simulink model "Sim_Ideal"  (R2017b)
settings: Solver=FixedStepAuto  StartTime=0.0  StopTime=t_total  FixedStep=1e-6  MaxStep=1e-4  RelTol=1e-3
values from neighbouring files (symbols this model uses):
  C21 = 100e-6    (= 0.0001)    [main_simu.m]
  C22 = 100e-6    (= 0.0001)    [main_simu.m]
  C23 = 220e-6    (= 0.00022)    [main_simu.m]
  C24 = 330e-6    (= 0.00033)    [main_simu.m]
  L41 = 10e-3    (= 0.01)    [main_simu.m]
  L42 = 10e-3    (= 0.01)    [main_simu.m]
  L43 = 10e-3    (= 0.01)    [main_simu.m]
  L44 = 100e-3    (= 0.1)    [main_simu.m]
  L61 = 1e-3    (= 0.001)    [main_simu.m]
  L62 = 1e-3    (= 0.001)    [main_simu.m]
  L63 = 1e-3    (= 0.001)    [main_simu.m]
  L64 = 1e-3    (= 0.001)    [main_simu.m]
  R21 = 2e3    (= 2000)    [main_simu.m]
  R22 = 1e3    (= 1000)    [main_simu.m]
  R23 = 500    [main_simu.m]
  R24 = 300    [main_simu.m]
  R31 = 2.5    [main_simu.m]
  R32 = 5    [main_simu.m]
  R33 = 8    [main_simu.m]
  R34 = 10    [main_simu.m]
  R41 = 10    [main_simu.m]
  R42 = 20    [main_simu.m]
  R43 = 30    [main_simu.m]
  R44 = 30    [main_simu.m]
  R51 = 10    [main_simu.m]
  R52 = 12    [main_simu.m]
  R53 = 15    [main_simu.m]
  R54 = 20    [main_simu.m]
  R61 = 10    [main_simu.m]
  R62 = 5    [main_simu.m]
  R63 = 30    [main_simu.m]
  R64 = 105    [main_simu.m]
  R71 = 5    [main_simu.m]
  R72 = 10    [main_simu.m]
  R73 = 20    [main_simu.m]
  R74 = 50    [main_simu.m]
  sim_off = sim_on    [double.m]    (also in fourfold.m; individual.m; main_simu.m; quintuple.m)
  sim_on = 50*ones(1,28)    [double.m]    (also in fourfold.m; individual.m; main_simu.m = 50*ones(1,num_cargas); quintuple.m)
  Valpha5 = 60    [main_simu.m]
  Valpha6 = 60    [main_simu.m]
undefined symbols (not defined in the file or in its folder): J, Laq, Lse, R, Ra, Rse, SEIP4, SEVP4, wm0, wmo
libraries: powerlib x204, simulink x72
(part 1 of 2)
settings Model: Creator=USUARIO  LastModifiedBy=USUARIO
settings SolverCC: DecoupledContinuousIntegration=on

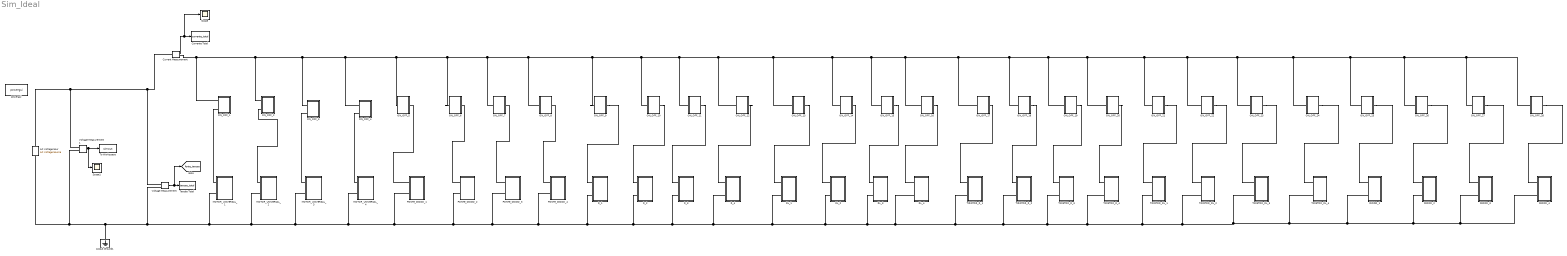
== system Sim_Ideal ==
  AC Voltage Sour : powerlib/Electrical Sources/AC Voltage Source  Amplitude=180  Phase=0  Frequency=60  SampleTime=0  Measurements=None  BusType=swing  Pref=10e3  Qref=0  Qmin=-inf  Qmax=+inf
  Corrente Total : ToWorkspace  VariableName=corrente_total  SampleTime=-1
  Current Measurement : powerlib/Measurements/Current Measurement  PhasorSimulation=off  OutputType=Complex  PSBequivalent=0
  DIODO_1 : Subsystem
  DIODO_2 : Subsystem
  DIODO_3 : Subsystem
  DIODO_4 : Subsystem
  MOTOR_UNIVERSAL_1 : Subsystem
  MOTOR_UNIVERSAL_2 : Subsystem
  MOTOR_UNIVERSAL_3 : Subsystem
  MOTOR_UNIVERSAL_4 : Subsystem
  ON_OFF_1 : Subsystem
  ON_OFF_10 : Subsystem
  ON_OFF_11 : Subsystem
  ON_OFF_12 : Subsystem
  ON_OFF_13 : Subsystem
  ON_OFF_14 : Subsystem
  ON_OFF_15 : Subsystem
  ON_OFF_16 : Subsystem
  ON_OFF_17 : Subsystem
  ON_OFF_18 : Subsystem
  ON_OFF_19 : Subsystem
  ON_OFF_2 : Subsystem
  ON_OFF_20 : Subsystem
  ON_OFF_21 : Subsystem
  ON_OFF_22 : Subsystem
  ON_OFF_23 : Subsystem
  ON_OFF_24 : Subsystem
  ON_OFF_25 : Subsystem
  ON_OFF_26 : Subsystem
  ON_OFF_27 : Subsystem
  ON_OFF_28 : Subsystem
  ON_OFF_3 : Subsystem
  ON_OFF_4 : Subsystem
  ON_OFF_5 : Subsystem
  ON_OFF_6 : Subsystem
  ON_OFF_7 : Subsystem
  ON_OFF_8 : Subsystem
  ON_OFF_9 : Subsystem
  PONTE_DIODO_1 : Subsystem
  PONTE_DIODO_2 : Subsystem
  PONTE_DIODO_3 : Subsystem
  PONTE_DIODO_4 : Subsystem
  RL_1 : Subsystem
  RL_2 : Subsystem
  RL_3 : Subsystem
  RL_4 : Subsystem
  R_1 : Subsystem
  R_2 : Subsystem
  R_3 : Subsystem
  R_4 : Subsystem
  Scope : Scope
  Scope1 : Scope
  TIRISTOR_RL_1 : Subsystem
  TIRISTOR_RL_2 : Subsystem
  TIRISTOR_RL_3 : Subsystem
  TIRISTOR_RL_4 : Subsystem
  TIRISTOR_R_1 : Subsystem
  TIRISTOR_R_2 : Subsystem
  TIRISTOR_R_3 : Subsystem
  TIRISTOR_R_4 : Subsystem
  Tensão Total : ToWorkspace  VariableName=tensao_total  SampleTime=-1
  To Workspace : ToWorkspace  VariableName=simout  SampleTime=-1
  Voltage Measurement : powerlib/Measurements/Voltage Measurement  PhasorSimulation=off  OutputType=Complex  PSBequivalent=0
  Voltage Measurement1 : powerlib/Measurements/Voltage Measurement  PhasorSimulation=off  OutputType=Complex  PSBequivalent=0
  output Ground1 : powerlib/Elements/Ground  LConnTagsString=a
  powergui : powerlib/powergui  Priority=1  SimulationMode=Discrete  SampleTime=1e-6  frequency=60  Iterations=100  frequencyindice=0  Pbase=100e6  ErrMax=1e-4  UnitsV=kV  UnitsW=MW  buscounter=0  FunctionMessages=off  echomessages=off  EnableUseOfTLC=off  CurrentSourceSwitches=off  DisableSnubberDevices=off  DisableRonSwitches=off  DisableVfSwitches=off  DisplayEquations=off  SolverType=Tustin/Backward Euler (TBE)  Interpol=off  ExternalGateDelay=off  methode=off  Ts=100  x0status=blocks  SPID=off  SwTol=0  HookPort=off  RestoreLinks=warning  ResistiveCurrentMeasurement=off  Frange=[0:2:500]  Ylog=off  Xlog=on  ShowGrid=off  save=off  variable=ZData  structure=0  ZoomFFT=off  StartTime=0.0  cycles=1  DisplayStyle=1  fundamental=60  FreqAxis=off  MaxFrequency=1000  frequencyindicesteady=1  RmsSteady=1  display=off
  tag scope: fonte_tensao=global
  wires:
  Current Measurement/1 -> Scope/1, Corrente Total/1
  Voltage Measurement/1 -> [fonte_tensao], Tensão Total/1
  Voltage Measurement1/1 -> Scope1/1, To Workspace/1
  connections:
  AC Voltage Sour/LConn1 -- Voltage Measurement1/LConn2 -- output Ground1/LConn1 -- Voltage Measurement/LConn2 -- MOTOR_UNIVERSAL_1/LConn2 -- MOTOR_UNIVERSAL_2/LConn2 -- MOTOR_UNIVERSAL_3/LConn2 -- MOTOR_UNIVERSAL_4/LConn2 -- PONTE_DIODO_4/LConn2 -- R_1/LConn2 -- R_4/LConn2 -- RL_4/LConn2 -- TIRISTOR_R_2/LConn2 -- TIRISTOR_RL_2/LConn2 -- DIODO_3/LConn2 -- DIODO_4/LConn2 -- DIODO_2/LConn2 -- DIODO_1/LConn2 -- TIRISTOR_RL_4/LConn2 -- TIRISTOR_RL_3/LConn2 -- TIRISTOR_RL_1/LConn2 -- TIRISTOR_R_4/LConn2 -- TIRISTOR_R_3/LConn2 -- TIRISTOR_R_1/LConn2 -- RL_3/LConn2 -- RL_2/LConn2 -- RL_1/LConn2 -- R_3/LConn2 -- R_2/LConn2 -- PONTE_DIODO_3/LConn2 -- PONTE_DIODO_2/LConn2 -- PONTE_DIODO_1/LConn2
  Voltage Measurement1/LConn1 -- Current Measurement/LConn1 -- Voltage Measurement/LConn1 -- AC Voltage Sour/RConn1
  MOTOR_UNIVERSAL_1/LConn1 -- ON_OFF_1/LConn2
  PONTE_DIODO_1/LConn1 -- ON_OFF_5/RConn1
  ON_OFF_9/RConn1 -- R_1/LConn1
  ON_OFF_13/RConn1 -- RL_1/LConn1
  ON_OFF_17/RConn1 -- TIRISTOR_R_1/LConn1
  ON_OFF_21/RConn1 -- TIRISTOR_RL_1/LConn1
  ON_OFF_14/RConn1 -- RL_2/LConn1
  ON_OFF_15/RConn1 -- RL_3/LConn1
  ON_OFF_16/RConn1 -- RL_4/LConn1
  ON_OFF_18/RConn1 -- TIRISTOR_R_2/LConn1
  ON_OFF_19/RConn1 -- TIRISTOR_R_3/LConn1
  ON_OFF_20/RConn1 -- TIRISTOR_R_4/LConn1
  ON_OFF_22/RConn1 -- TIRISTOR_RL_2/LConn1
  ON_OFF_23/RConn1 -- TIRISTOR_RL_3/LConn1
  ON_OFF_24/RConn1 -- TIRISTOR_RL_4/LConn1
  ON_OFF_10/RConn1 -- R_2/LConn1
  ON_OFF_11/RConn1 -- R_3/LConn1
  ON_OFF_12/RConn1 -- R_4/LConn1
  PONTE_DIODO_2/LConn1 -- ON_OFF_6/RConn1
  PONTE_DIODO_3/LConn1 -- ON_OFF_7/RConn1
  PONTE_DIODO_4/LConn1 -- ON_OFF_8/RConn1
  ON_OFF_25/RConn1 -- DIODO_1/LConn1
  ON_OFF_26/RConn1 -- DIODO_2/LConn1
  ON_OFF_27/RConn1 -- DIODO_3/LConn1
  ON_OFF_28/RConn1 -- DIODO_4/LConn1
  MOTOR_UNIVERSAL_2/LConn1 -- ON_OFF_2/LConn2
  MOTOR_UNIVERSAL_4/LConn1 -- ON_OFF_4/LConn2
  MOTOR_UNIVERSAL_3/LConn1 -- ON_OFF_3/LConn2
  ON_OFF_28/LConn1 -- ON_OFF_27/LConn1 -- ON_OFF_26/LConn1 -- ON_OFF_25/LConn1 -- ON_OFF_24/LConn1 -- ON_OFF_23/LConn1 -- ON_OFF_22/LConn1 -- ON_OFF_21/LConn1 -- ON_OFF_20/LConn1 -- ON_OFF_19/LConn1 -- ON_OFF_18/LConn1 -- ON_OFF_17/LConn1 -- ON_OFF_16/LConn1 -- ON_OFF_15/LConn1 -- ON_OFF_14/LConn1 -- ON_OFF_13/LConn1 -- ON_OFF_12/LConn1 -- ON_OFF_11/LConn1 -- ON_OFF_10/LConn1 -- ON_OFF_9/LConn1 -- ON_OFF_8/LConn1 -- ON_OFF_7/LConn1 -- ON_OFF_6/LConn1 -- Current Measurement/RConn1 -- ON_OFF_1/LConn1 -- ON_OFF_2/LConn1 -- ON_OFF_3/LConn1 -- ON_OFF_4/LConn1 -- ON_OFF_5/LConn1

== system Sim_Ideal/DIODO_1 ==
  note: LOAD
  Diode : powerlib/Power Electronics/Diode  Ron=0.001  Lon=0  Vf=0.8  IC=0  UseSnubber=0  Rs=500  Cs=250e-9  Measurements=off
  Ground2 : powerlib/Elements/Ground  LConnTagsString=a
  Scope : Scope
  Scope1 : Scope
  Series RLC Branch : powerlib/Elements/Series RLC Branch  LConnTagsString=__new0  RConnTagsString=__new0  BranchType=R  Resistance=R71  Inductance=1e-3  SetiL0=off  InitialCurrent=0  Capacitance=1e-6  Setx0=off  InitialVoltage=0  Measurements=None
  To Workspace1 : ToWorkspace  VariableName=corrente_diodo_1  SampleTime=-1
  To Workspace4 : ToWorkspace  VariableName=tensao_diodo_1  SampleTime=-1
  V_Load : powerlib/Measurements/Voltage Measurement  PhasorSimulation=off  OutputType=Complex  PSBequivalent=0
  i_Load : powerlib/Measurements/Current Measurement  Tag=PoWeRsYsTeMmEaSuReMeNt  PhasorSimulation=off  OutputType=Magnitude  PSBequivalent=0
  Conn1 : PMIOPort  Port=1  Side=Left
  Conn2 : PMIOPort  Port=2  Side=Left
  wires:
  i_Load/1 -> To Workspace1/1, Scope1/1
  V_Load/1 -> To Workspace4/1, Scope/1
  connections:
  Series RLC Branch/LConn1 -- Diode/RConn1 -- V_Load/LConn1
  V_Load/LConn2 -- Series RLC Branch/RConn1 -- Conn2/RConn1 -- Ground2/LConn1
  i_Load/RConn1 -- Diode/LConn1
  i_Load/LConn1 -- Conn1/RConn1

== system Sim_Ideal/DIODO_2 ==
  note: LOAD
  Diode : powerlib/Power Electronics/Diode  Ron=0.001  Lon=0  Vf=0.8  IC=0  UseSnubber=0  Rs=500  Cs=250e-9  Measurements=off
  Ground2 : powerlib/Elements/Ground  LConnTagsString=a
  Scope : Scope
  Scope1 : Scope
  Series RLC Branch : powerlib/Elements/Series RLC Branch  LConnTagsString=__new0  RConnTagsString=__new0  BranchType=R  Resistance=R72  Inductance=1e-3  SetiL0=off  InitialCurrent=0  Capacitance=1e-6  Setx0=off  InitialVoltage=0  Measurements=None
  To Workspace1 : ToWorkspace  VariableName=corrente_diodo_2  SampleTime=-1
  To Workspace4 : ToWorkspace  VariableName=tensao_diodo_2  SampleTime=-1
  V_Load : powerlib/Measurements/Voltage Measurement  PhasorSimulation=off  OutputType=Complex  PSBequivalent=0
  i_Load : powerlib/Measurements/Current Measurement  Tag=PoWeRsYsTeMmEaSuReMeNt  PhasorSimulation=off  OutputType=Magnitude  PSBequivalent=0
  Conn1 : PMIOPort  Port=1  Side=Left
  Conn2 : PMIOPort  Port=2  Side=Left
  wires:
  i_Load/1 -> To Workspace1/1, Scope1/1
  V_Load/1 -> To Workspace4/1, Scope/1
  connections:
  Series RLC Branch/LConn1 -- V_Load/LConn1 -- Diode/RConn1
  Series RLC Branch/RConn1 -- V_Load/LConn2 -- Ground2/LConn1 -- Conn2/RConn1
  i_Load/RConn1 -- Diode/LConn1
  i_Load/LConn1 -- Conn1/RConn1

== system Sim_Ideal/DIODO_3 ==
  note: LOAD
  Diode : powerlib/Power Electronics/Diode  Ron=0.001  Lon=0  Vf=0.8  IC=0  UseSnubber=0  Rs=500  Cs=250e-9  Measurements=off
  Ground2 : powerlib/Elements/Ground  LConnTagsString=a
  Scope : Scope
  Scope1 : Scope
  Series RLC Branch : powerlib/Elements/Series RLC Branch  LConnTagsString=__new0  RConnTagsString=__new0  BranchType=R  Resistance=R73  Inductance=1e-3  SetiL0=off  InitialCurrent=0  Capacitance=1e-6  Setx0=off  InitialVoltage=0  Measurements=None
  To Workspace1 : ToWorkspace  VariableName=corrente_diodo_3  SampleTime=-1
  To Workspace4 : ToWorkspace  VariableName=tensao_diodo_3  SampleTime=-1
  V_Load : powerlib/Measurements/Voltage Measurement  PhasorSimulation=off  OutputType=Complex  PSBequivalent=0
  i_Load : powerlib/Measurements/Current Measurement  Tag=PoWeRsYsTeMmEaSuReMeNt  PhasorSimulation=off  OutputType=Magnitude  PSBequivalent=0
  Conn1 : PMIOPort  Port=1  Side=Left
  Conn2 : PMIOPort  Port=2  Side=Left
  wires:
  i_Load/1 -> To Workspace1/1, Scope1/1
  V_Load/1 -> To Workspace4/1, Scope/1
  connections:
  Series RLC Branch/LConn1 -- V_Load/LConn1 -- Diode/RConn1
  Series RLC Branch/RConn1 -- V_Load/LConn2 -- Ground2/LConn1 -- Conn2/RConn1
  i_Load/RConn1 -- Diode/LConn1
  i_Load/LConn1 -- Conn1/RConn1

== system Sim_Ideal/DIODO_4 ==
  note: LOAD
  Diode : powerlib/Power Electronics/Diode  Ron=0.001  Lon=0  Vf=0.8  IC=0  UseSnubber=0  Rs=500  Cs=250e-9  Measurements=off
  Ground2 : powerlib/Elements/Ground  LConnTagsString=a
  Scope : Scope
  Scope1 : Scope
  Series RLC Branch : powerlib/Elements/Series RLC Branch  LConnTagsString=__new0  RConnTagsString=__new0  BranchType=R  Resistance=R74  Inductance=1e-3  SetiL0=off  InitialCurrent=0  Capacitance=1e-6  Setx0=off  InitialVoltage=0  Measurements=None
  To Workspace1 : ToWorkspace  VariableName=corrente_diodo_4  SampleTime=-1
  To Workspace4 : ToWorkspace  VariableName=tensao_diodo_4  SampleTime=-1
  V_Load : powerlib/Measurements/Voltage Measurement  PhasorSimulation=off  OutputType=Complex  PSBequivalent=0
  i_Load : powerlib/Measurements/Current Measurement  Tag=PoWeRsYsTeMmEaSuReMeNt  PhasorSimulation=off  OutputType=Magnitude  PSBequivalent=0
  Conn1 : PMIOPort  Port=1  Side=Left
  Conn2 : PMIOPort  Port=2  Side=Left
  wires:
  i_Load/1 -> To Workspace1/1, Scope1/1
  V_Load/1 -> To Workspace4/1, Scope/1
  connections:
  Series RLC Branch/LConn1 -- V_Load/LConn1 -- Diode/RConn1
  Series RLC Branch/RConn1 -- V_Load/LConn2 -- Ground2/LConn1 -- Conn2/RConn1
  i_Load/RConn1 -- Diode/LConn1
  i_Load/LConn1 -- Conn1/RConn1

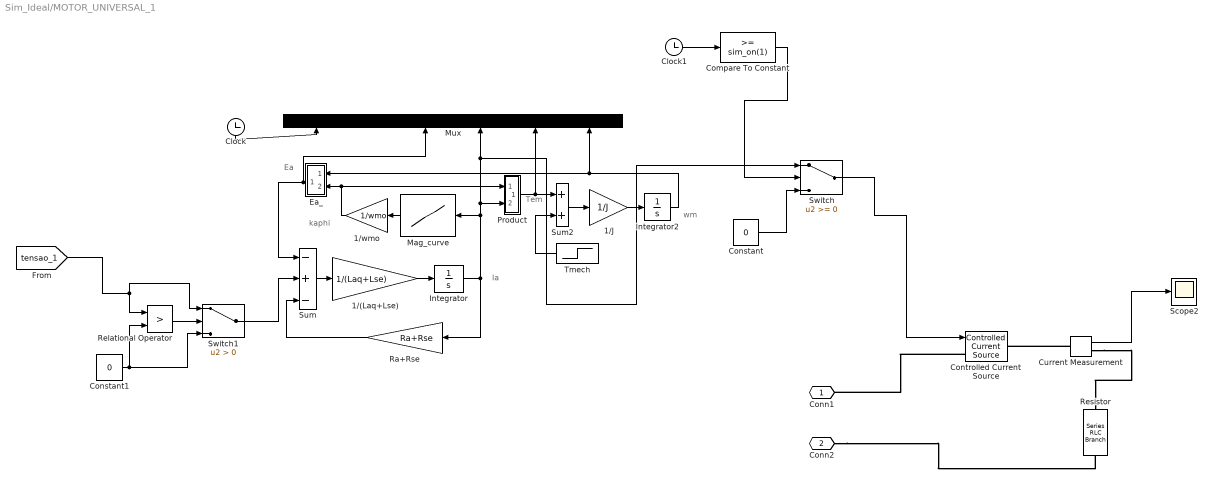
== system Sim_Ideal/MOTOR_UNIVERSAL_1 ==
  note: kaphi
  note: Tem
  note: Ea
  note: wm
  note: Ia
  1/(Laq+Lse) : Gain  Gain=1/(Laq+Lse)  SaturateOnIntegerOverflow=on  OutDataTypeStr=Inherit: Same as input  ParamDataTypeStr=Inherit: Same as input
  1/J : Gain  Gain=1/J  SaturateOnIntegerOverflow=on  OutDataTypeStr=Inherit: Same as input  ParamDataTypeStr=Inherit: Same as input
  1/wmo : Gain  Gain=1/wmo  SaturateOnIntegerOverflow=on  OutDataTypeStr=Inherit: Same as input  ParamDataTypeStr=Inherit: Same as input
  Clock : Clock
  Clock1 : Clock
  Compare To Constant : simulink/Logic and Bit Operations/Compare To Constant  relop=>=  const=sim_on(1)  OutDataTypeStr=boolean
  Constant : Constant  Value=0
  Constant1 : Constant  Value=0
  Controlled Current Source : powerlib/Electrical Sources/Controlled Current Source  Initialize=on  Source_Type=AC  Amplitude=0  Phase=0  Frequency=0  Measurements=None
  Current Measurement : powerlib/Measurements/Current Measurement  PhasorSimulation=off  OutputType=Complex  PSBequivalent=0
  Ea_ : Subsystem  mask(Dot Product){}
      mask help:
      | Inner (dot) product.
      | y=sum(u1.*u2)
      mask Help: Computes the inner (dot) product of the inputs: sum(u1.*u2).  The inputs are vectors of the same length. Output is a scalar.
      mask Display: disp('.\n')
  Integrator : Integrator
  Integrator2 : Integrator  InitialCondition=wm0
  Mag_curve : Lookup  InputValues=SEIP4  Table=SEVP4  SaturateOnIntegerOverflow=on
  Mux : Mux  Inputs=6
  Product : Subsystem  mask(Dot Product){}
      mask help:
      | Inner (dot) product.
      | y=sum(u1.*u2)
      mask Help: Computes the inner (dot) product of the inputs: sum(u1.*u2).  The inputs are vectors of the same length. Output is a scalar.
      mask Display: disp('.\n')
  Ra+Rse : Gain  Gain=Ra+Rse  SaturateOnIntegerOverflow=on  OutDataTypeStr=Inherit: Same as input  ParamDataTypeStr=Inherit: Same as input
  Relational Operator : RelationalOperator  Operator=>  OutDataTypeStr=boolean  RndMeth=Simplest
  Resistor : powerlib/Elements/Series RLC Branch  LConnTagsString=__new0  RConnTagsString=__new0  BranchType=R  Resistance=1e-15  Inductance=1e-3  SetiL0=off  InitialCurrent=0  Capacitance=1e-6  Setx0=off  InitialVoltage=0  Measurements=None
  Scope2 : Scope
  Sum : Sum  Inputs=-+-  SaturateOnIntegerOverflow=on  InputSameDT=on  OutDataTypeStr=Inherit: Same as first input
  Sum2 : Sum  SaturateOnIntegerOverflow=on  InputSameDT=on  OutDataTypeStr=Inherit: Same as first input
  Switch : Switch
  Switch1 : Switch  Criteria=u2 > Threshold
  Tmech : Step  Time=0  Before=-0.8  After=2
  Conn1 : PMIOPort  Port=1  Side=Left
  Conn2 : PMIOPort  Port=2  Side=Left
  wires:
  Ra+Rse/1 -> Sum/3
  1/J/1 -> Integrator2/1
  1/wmo/1 -> Ea_/2(in_2), Product/1(in_1)
  Current Measurement/1 -> Scope2/1
  Mag_curve/1 -> 1/wmo/1
  Sum/1 -> 1/(Laq+Lse)/1
  Sum2/1 -> 1/J/1
  1/(Laq+Lse)/1 -> Integrator/1
  Ea_/1(out_1) -> Mux/3, Sum/1
  Integrator2/1 -> Mux/6, Ea_/1(in_1)
  Tmech/1 -> Sum2/2
  Integrator/1 -> Switch/1, Mux/4, Product/2(in_2), Mag_curve/1, Ra+Rse/1
  Clock/1 -> Mux/1
  Product/1(out_1) -> Mux/5, Sum2/1
  Constant/1 -> Switch/3
  Compare To Constant/1 -> Switch/2
  Clock1/1 -> Compare To Constant/1
  Switch/1 -> Controlled Current Source/1
  Relational Operator/1 -> Switch1/2
  Constant1/1 -> Relational Operator/2, Switch1/3
  Switch1/1 -> Sum/2
  [tensao_1] -> Relational Operator/1, Switch1/1
  connections:
  Conn2/RConn1 -- Resistor/RConn1
  Controlled Current Source/LConn1 -- Conn1/RConn1
  Current Measurement/LConn1 -- Controlled Current Source/RConn1
  Current Measurement/RConn1 -- Resistor/LConn1

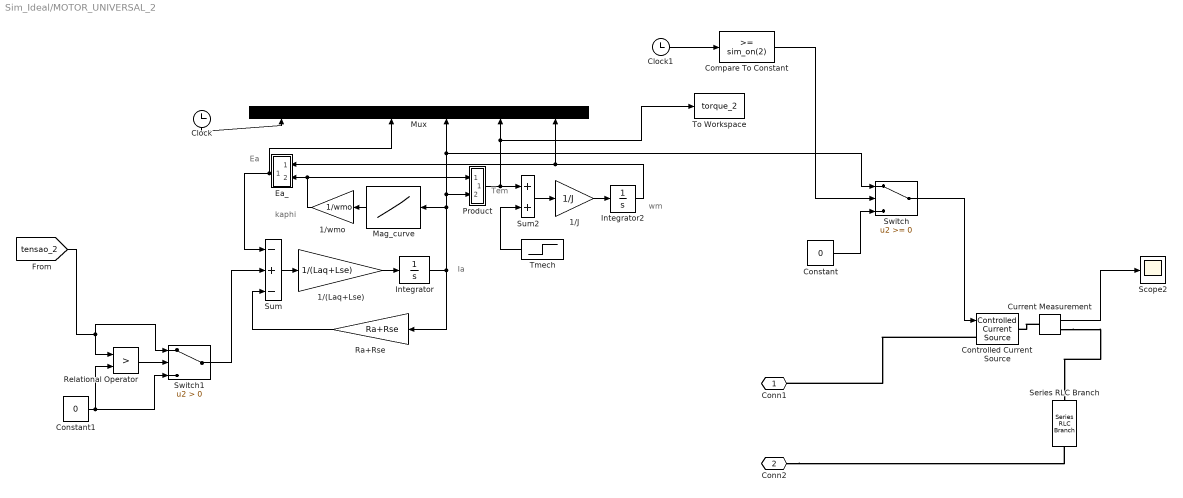
== system Sim_Ideal/MOTOR_UNIVERSAL_2 ==
  note: kaphi
  note: Tem
  note: Ea
  note: wm
  note: Ia
  1/(Laq+Lse) : Gain  Gain=1/(Laq+Lse)  SaturateOnIntegerOverflow=on  OutDataTypeStr=Inherit: Same as input  ParamDataTypeStr=Inherit: Same as input
  1/J : Gain  Gain=1/J  SaturateOnIntegerOverflow=on  OutDataTypeStr=Inherit: Same as input  ParamDataTypeStr=Inherit: Same as input
  1/wmo : Gain  Gain=1/wmo  SaturateOnIntegerOverflow=on  OutDataTypeStr=Inherit: Same as input  ParamDataTypeStr=Inherit: Same as input
  Clock : Clock
  Clock1 : Clock
  Compare To Constant : simulink/Logic and Bit Operations/Compare To Constant  relop=>=  const=sim_on(2)  OutDataTypeStr=boolean
  Constant : Constant  Value=0
  Constant1 : Constant  Value=0
  Controlled Current Source : powerlib/Electrical Sources/Controlled Current Source  Initialize=on  Source_Type=AC  Amplitude=0  Phase=0  Frequency=0  Measurements=None
  Current Measurement : powerlib/Measurements/Current Measurement  PhasorSimulation=off  OutputType=Complex  PSBequivalent=0
  Ea_ : Subsystem  mask(Dot Product){}
      mask help:
      | Inner (dot) product.
      | y=sum(u1.*u2)
      mask Help: Computes the inner (dot) product of the inputs: sum(u1.*u2).  The inputs are vectors of the same length. Output is a scalar.
      mask Display: disp('.\n')
  Integrator : Integrator
  Integrator2 : Integrator  InitialCondition=wm0
  Mag_curve : Lookup  InputValues=SEIP4  Table=SEVP4  SaturateOnIntegerOverflow=on
  Mux : Mux  Inputs=6
  Product : Subsystem  mask(Dot Product){}
      mask help:
      | Inner (dot) product.
      | y=sum(u1.*u2)
      mask Help: Computes the inner (dot) product of the inputs: sum(u1.*u2).  The inputs are vectors of the same length. Output is a scalar.
      mask Display: disp('.\n')
  Ra+Rse : Gain  Gain=Ra+Rse  SaturateOnIntegerOverflow=on  OutDataTypeStr=Inherit: Same as input  ParamDataTypeStr=Inherit: Same as input
  Relational Operator : RelationalOperator  Operator=>  OutDataTypeStr=boolean  RndMeth=Simplest
  Scope2 : Scope
  Series RLC Branch : powerlib/Elements/Series RLC Branch  LConnTagsString=__new0  RConnTagsString=__new0  BranchType=R  Resistance=1e-15  Inductance=1e-3  SetiL0=off  InitialCurrent=0  Capacitance=1e-6  Setx0=off  InitialVoltage=0  Measurements=None
  Sum : Sum  Inputs=-+-  SaturateOnIntegerOverflow=on  InputSameDT=on  OutDataTypeStr=Inherit: Same as first input
  Sum2 : Sum  SaturateOnIntegerOverflow=on  InputSameDT=on  OutDataTypeStr=Inherit: Same as first input
  Switch : Switch
  Switch1 : Switch  Criteria=u2 > Threshold
  Tmech : Step  Time=0  Before=-0.8
  To Workspace : ToWorkspace  VariableName=torque_2  SaveFormat=Timeseries  SampleTime=-1
  Conn1 : PMIOPort  Port=1  Side=Left
  Conn2 : PMIOPort  Port=2  Side=Left
  wires:
  Ra+Rse/1 -> Sum/3
  1/J/1 -> Integrator2/1
  1/wmo/1 -> Ea_/2(in_2), Product/1(in_1)
  Current Measurement/1 -> Scope2/1
  Mag_curve/1 -> 1/wmo/1
  Sum/1 -> 1/(Laq+Lse)/1
  Sum2/1 -> 1/J/1
  1/(Laq+Lse)/1 -> Integrator/1
  Ea_/1(out_1) -> Mux/3, Sum/1
  Integrator2/1 -> Mux/6, Ea_/1(in_1)
  Tmech/1 -> Sum2/2
  Integrator/1 -> Mux/4, Switch/1, Product/2(in_2), Mag_curve/1, Ra+Rse/1
  Clock/1 -> Mux/1
  Product/1(out_1) -> To Workspace/1, Mux/5, Sum2/1
  Switch/1 -> Controlled Current Source/1
  Constant/1 -> Switch/3
  Compare To Constant/1 -> Switch/2
  Clock1/1 -> Compare To Constant/1
  Constant1/1 -> Relational Operator/2, Switch1/3
  Relational Operator/1 -> Switch1/2
  Switch1/1 -> Sum/2
  [tensao_2] -> Relational Operator/1, Switch1/1
  connections:
  Conn2/RConn1 -- Series RLC Branch/RConn1
  Controlled Current Source/LConn1 -- Conn1/RConn1
  Current Measurement/LConn1 -- Controlled Current Source/RConn1
  Current Measurement/RConn1 -- Series RLC Branch/LConn1

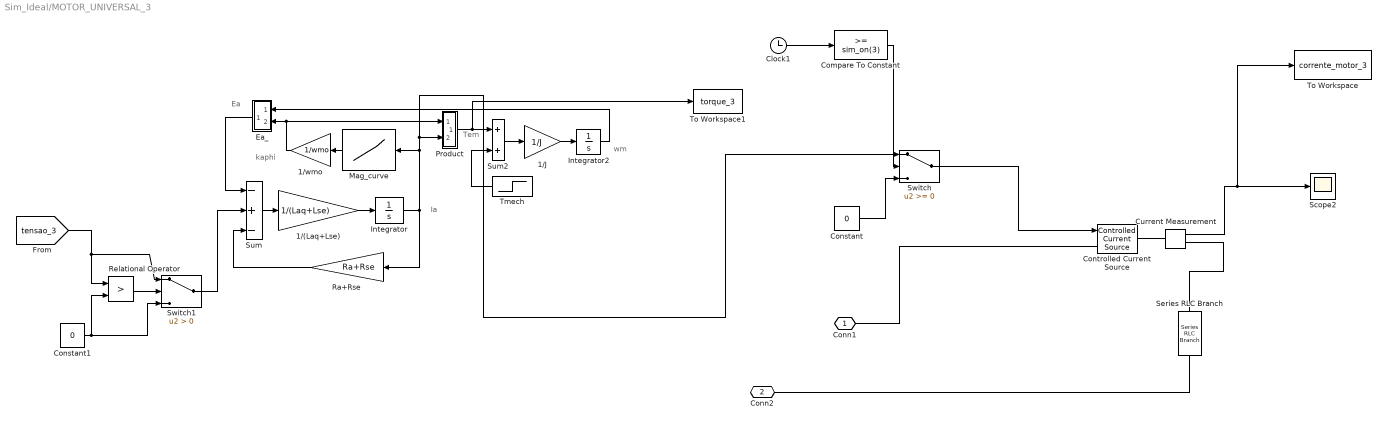
== system Sim_Ideal/MOTOR_UNIVERSAL_3 ==
  note: kaphi
  note: Tem
  note: Ea
  note: wm
  note: Ia
  1/(Laq+Lse) : Gain  Gain=1/(Laq+Lse)  SaturateOnIntegerOverflow=on  OutDataTypeStr=Inherit: Same as input  ParamDataTypeStr=Inherit: Same as input
  1/J : Gain  Gain=1/J  SaturateOnIntegerOverflow=on  OutDataTypeStr=Inherit: Same as input  ParamDataTypeStr=Inherit: Same as input
  1/wmo : Gain  Gain=1/wmo  SaturateOnIntegerOverflow=on  OutDataTypeStr=Inherit: Same as input  ParamDataTypeStr=Inherit: Same as input
  Clock1 : Clock
  Compare To Constant : simulink/Logic and Bit Operations/Compare To Constant  relop=>=  const=sim_on(3)  OutDataTypeStr=boolean
  Constant : Constant  Value=0
  Constant1 : Constant  Value=0
  Controlled Current Source : powerlib/Electrical Sources/Controlled Current Source  Initialize=on  Source_Type=AC  Amplitude=0  Phase=0  Frequency=0  Measurements=None
  Current Measurement : powerlib/Measurements/Current Measurement  PhasorSimulation=off  OutputType=Complex  PSBequivalent=0
  Ea_ : Subsystem  mask(Dot Product){}
      mask help:
      | Inner (dot) product.
      | y=sum(u1.*u2)
      mask Help: Computes the inner (dot) product of the inputs: sum(u1.*u2).  The inputs are vectors of the same length. Output is a scalar.
      mask Display: disp('.\n')
  Integrator : Integrator
  Integrator2 : Integrator  InitialCondition=wm0
  Mag_curve : Lookup  InputValues=SEIP4  Table=SEVP4  SaturateOnIntegerOverflow=on
  Product : Subsystem  mask(Dot Product){}
      mask help:
      | Inner (dot) product.
      | y=sum(u1.*u2)
      mask Help: Computes the inner (dot) product of the inputs: sum(u1.*u2).  The inputs are vectors of the same length. Output is a scalar.
      mask Display: disp('.\n')
  Ra+Rse : Gain  Gain=Ra+Rse  SaturateOnIntegerOverflow=on  OutDataTypeStr=Inherit: Same as input  ParamDataTypeStr=Inherit: Same as input
  Relational Operator : RelationalOperator  Operator=>  OutDataTypeStr=boolean  RndMeth=Simplest
  Scope2 : Scope
  Series RLC Branch : powerlib/Elements/Series RLC Branch  LConnTagsString=__new0  RConnTagsString=__new0  BranchType=R  Resistance=1e-100  Inductance=1e-3  SetiL0=off  InitialCurrent=0  Capacitance=1e-6  Setx0=off  InitialVoltage=0  Measurements=None
  Sum : Sum  Inputs=-+-  SaturateOnIntegerOverflow=on  InputSameDT=on  OutDataTypeStr=Inherit: Same as first input
  Sum2 : Sum  SaturateOnIntegerOverflow=on  InputSameDT=on  OutDataTypeStr=Inherit: Same as first input
  Switch : Switch
  Switch1 : Switch  Criteria=u2 > Threshold
  Tmech : Step  Time=0  Before=-0.8  After=-0.1
  To Workspace : ToWorkspace  VariableName=corrente_motor_3  SampleTime=-1
  To Workspace1 : ToWorkspace  VariableName=torque_3  SaveFormat=Timeseries  SampleTime=-1
  Conn1 : PMIOPort  Port=1  Side=Left
  Conn2 : PMIOPort  Port=2  Side=Left
  wires:
  Ra+Rse/1 -> Sum/3
  1/J/1 -> Integrator2/1
  1/wmo/1 -> Ea_/2(in_2), Product/1(in_1)
  Current Measurement/1 -> To Workspace/1, Scope2/1
  Mag_curve/1 -> 1/wmo/1
  Sum/1 -> 1/(Laq+Lse)/1
  Sum2/1 -> 1/J/1
  1/(Laq+Lse)/1 -> Integrator/1
  Ea_/1(out_1) -> Sum/1
  Integrator2/1 -> Ea_/1(in_1)
  Tmech/1 -> Sum2/2
  Integrator/1 -> Switch/1, Product/2(in_2), Mag_curve/1, Ra+Rse/1
  Product/1(out_1) -> To Workspace1/1, Sum2/1
  Switch/1 -> Controlled Current Source/1
  Clock1/1 -> Compare To Constant/1
  Compare To Constant/1 -> Switch/2
  Constant/1 -> Switch/3
  Relational Operator/1 -> Switch1/2
  Constant1/1 -> Relational Operator/2, Switch1/3
  Switch1/1 -> Sum/2
  [tensao_3] -> Relational Operator/1, Switch1/1
  connections:
  Conn2/RConn1 -- Series RLC Branch/RConn1
  Current Measurement/LConn1 -- Controlled Current Source/RConn1
  Current Measurement/RConn1 -- Series RLC Branch/LConn1
  Conn1/RConn1 -- Controlled Current Source/LConn1

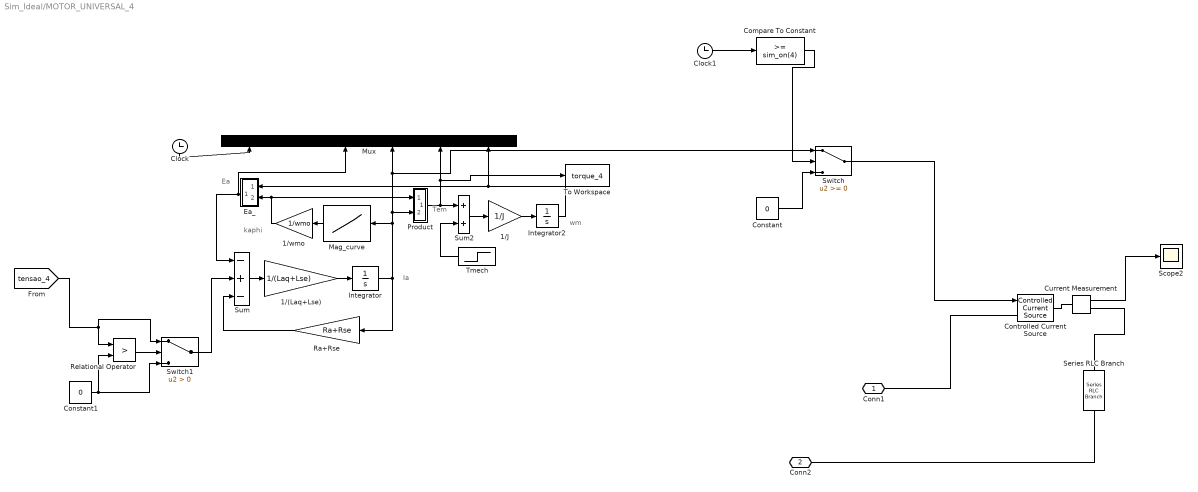
== system Sim_Ideal/MOTOR_UNIVERSAL_4 ==
  note: kaphi
  note: Tem
  note: Ea
  note: wm
  note: Ia
  1/(Laq+Lse) : Gain  Gain=1/(Laq+Lse)  SaturateOnIntegerOverflow=on  OutDataTypeStr=Inherit: Same as input  ParamDataTypeStr=Inherit: Same as input
  1/J : Gain  Gain=1/J  SaturateOnIntegerOverflow=on  OutDataTypeStr=Inherit: Same as input  ParamDataTypeStr=Inherit: Same as input
  1/wmo : Gain  Gain=1/wmo  SaturateOnIntegerOverflow=on  OutDataTypeStr=Inherit: Same as input  ParamDataTypeStr=Inherit: Same as input
  Clock : Clock
  Clock1 : Clock
  Compare To Constant : simulink/Logic and Bit Operations/Compare To Constant  relop=>=  const=sim_on(4)  OutDataTypeStr=boolean
  Constant : Constant  Value=0
  Constant1 : Constant  Value=0
  Controlled Current Source : powerlib/Electrical Sources/Controlled Current Source  Initialize=on  Source_Type=AC  Amplitude=0  Phase=0  Frequency=0  Measurements=None
  Current Measurement : powerlib/Measurements/Current Measurement  PhasorSimulation=off  OutputType=Complex  PSBequivalent=0
  Ea_ : Subsystem  mask(Dot Product){}
      mask help:
      | Inner (dot) product.
      | y=sum(u1.*u2)
      mask Help: Computes the inner (dot) product of the inputs: sum(u1.*u2).  The inputs are vectors of the same length. Output is a scalar.
      mask Display: disp('.\n')
  Integrator : Integrator
  Integrator2 : Integrator  InitialCondition=wm0
  Mag_curve : Lookup  InputValues=SEIP4  Table=SEVP4  SaturateOnIntegerOverflow=on
  Mux : Mux  Inputs=6
  Product : Subsystem  mask(Dot Product){}
      mask help:
      | Inner (dot) product.
      | y=sum(u1.*u2)
      mask Help: Computes the inner (dot) product of the inputs: sum(u1.*u2).  The inputs are vectors of the same length. Output is a scalar.
      mask Display: disp('.\n')
  Ra+Rse : Gain  Gain=Ra+Rse  SaturateOnIntegerOverflow=on  OutDataTypeStr=Inherit: Same as input  ParamDataTypeStr=Inherit: Same as input
  Relational Operator : RelationalOperator  Operator=>  OutDataTypeStr=boolean  RndMeth=Simplest
  Scope2 : Scope
  Series RLC Branch : powerlib/Elements/Series RLC Branch  LConnTagsString=__new0  RConnTagsString=__new0  BranchType=R  Resistance=1e-15  Inductance=1e-3  SetiL0=off  InitialCurrent=0  Capacitance=1e-6  Setx0=off  InitialVoltage=0  Measurements=None
  Sum : Sum  Inputs=-+-  SaturateOnIntegerOverflow=on  InputSameDT=on  OutDataTypeStr=Inherit: Same as first input
  Sum2 : Sum  SaturateOnIntegerOverflow=on  InputSameDT=on  OutDataTypeStr=Inherit: Same as first input
  Switch : Switch
  Switch1 : Switch  Criteria=u2 > Threshold
  Tmech : Step  Time=0  Before=-0.8  After=0.5
  To Workspace : ToWorkspace  VariableName=torque_4  SaveFormat=Timeseries  SampleTime=-1
  Conn1 : PMIOPort  Port=1  Side=Left
  Conn2 : PMIOPort  Port=2  Side=Left
  wires:
  Ra+Rse/1 -> Sum/3
  1/J/1 -> Integrator2/1
  1/wmo/1 -> Ea_/2(in_2), Product/1(in_1)
  Current Measurement/1 -> Scope2/1
  Mag_curve/1 -> 1/wmo/1
  Sum/1 -> 1/(Laq+Lse)/1
  Sum2/1 -> 1/J/1
  1/(Laq+Lse)/1 -> Integrator/1
  Ea_/1(out_1) -> Mux/3, Sum/1
  Integrator2/1 -> Mux/6, Ea_/1(in_1)
  Tmech/1 -> Sum2/2
  Integrator/1 -> Switch/1, Mux/4, Product/2(in_2), Mag_curve/1, Ra+Rse/1
  Clock/1 -> Mux/1
  Product/1(out_1) -> To Workspace/1, Mux/5, Sum2/1
  Constant/1 -> Switch/3
  Compare To Constant/1 -> Switch/2
  Clock1/1 -> Compare To Constant/1
  Switch/1 -> Controlled Current Source/1
  Relational Operator/1 -> Switch1/2
  Constant1/1 -> Relational Operator/2, Switch1/3
  Switch1/1 -> Sum/2
  [tensao_4] -> Relational Operator/1, Switch1/1
  connections:
  Conn2/RConn1 -- Series RLC Branch/RConn1
  Controlled Current Source/LConn1 -- Conn1/RConn1
  Current Measurement/LConn1 -- Controlled Current Source/RConn1
  Current Measurement/RConn1 -- Series RLC Branch/LConn1

== system Sim_Ideal/ON_OFF_1 ==
  Clock1 : Clock
  Clock2 : Clock
  Clock3 : Clock
  Compare To Constant : simulink/Logic and Bit Operations/Compare To Constant  relop=>=  const=sim_on(1)  OutDataTypeStr=boolean
  Compare To Constant1 : simulink/Logic and Bit Operations/Compare To Constant  relop=>=  const=sim_off(1)  OutDataTypeStr=boolean
  Compare To Constant2 : simulink/Logic and Bit Operations/Compare To Constant  relop=>=  const=sim_on(1)  OutDataTypeStr=boolean
  Constant : Constant  Value=0
  Constant1 : Constant  Value=0
  Ideal Switch : powerlib/Power Electronics/Ideal Switch  Ron=0.001  Lon=0  IC=0  Rs=1e5  Cs=inf  Measurements=off
  Series RLC Branch : powerlib/Elements/Series RLC Branch  LConnTagsString=__new0  RConnTagsString=__new0  BranchType=R  Resistance=1e-10  Inductance=1e-3  SetiL0=off  InitialCurrent=0  Capacitance=1e-6  Setx0=off  InitialVoltage=0  Measurements=None
  Switch : Switch
  Switch1 : Switch
  Conn1 : PMIOPort  Port=1  Side=Left
  Conn2 : PMIOPort  Port=2  Side=Left
  tag scope: tensao_1=global
  wires:
  Switch1/1 -> [tensao_1]
  Constant/1 -> Switch/3
  Switch/1 -> Switch1/3
  Clock1/1 -> Compare To Constant/1
  Clock2/1 -> Compare To Constant1/1
  Compare To Constant1/1 -> Switch1/2
  [fonte_tensao] -> Switch/1
  Constant1/1 -> Switch1/1
  Compare To Constant/1 -> Switch/2
  Clock3/1 -> Compare To Constant2/1
  Compare To Constant2/1 -> Ideal Switch/1
  connections:
  Conn1/RConn1 -- Ideal Switch/LConn1
  Series RLC Branch/RConn1 -- Conn2/RConn1
  Ideal Switch/RConn1 -- Series RLC Branch/LConn1

== system Sim_Ideal/ON_OFF_10 ==
  Clock4 : Clock
  Compare To Constant2 : simulink/Logic and Bit Operations/Compare To Constant  relop=>=  const=sim_on(10)  OutDataTypeStr=boolean
  Compare To Constat3 : simulink/Logic and Bit Operations/Compare To Constant  relop=<=  const=sim_off(10)  OutDataTypeStr=boolean
  OFF2 : powerlib/Power Electronics/Ideal Switch  Ron=0.001  Lon=0  IC=0  Rs=1e5  Cs=inf  Measurements=off
  ON2 : powerlib/Power Electronics/Ideal Switch  Ron=0.001  Lon=0  IC=0  Rs=1e5  Cs=inf  Measurements=off
  Conn1 : PMIOPort  Port=1  Side=Left
  Conn2 : PMIOPort  Port=2  Side=Right
  wires:
  Compare To Constant2/1 -> ON2/1
  Compare To Constat3/1 -> OFF2/1
  Clock4/1 -> Compare To Constat3/1, Compare To Constant2/1
  connections:
  OFF2/RConn1 -- Conn2/RConn1
  ON2/RConn1 -- OFF2/LConn1
  ON2/LConn1 -- Conn1/RConn1

== system Sim_Ideal/ON_OFF_11 ==
  Clock4 : Clock
  Compare To Constant2 : simulink/Logic and Bit Operations/Compare To Constant  relop=>=  const=sim_on(11)  OutDataTypeStr=boolean
  Compare To Constat3 : simulink/Logic and Bit Operations/Compare To Constant  relop=<=  const=sim_off(11)  OutDataTypeStr=boolean
  OFF2 : powerlib/Power Electronics/Ideal Switch  Ron=0.001  Lon=0  IC=0  Rs=1e5  Cs=inf  Measurements=off
  ON2 : powerlib/Power Electronics/Ideal Switch  Ron=0.001  Lon=0  IC=0  Rs=1e5  Cs=inf  Measurements=off
  Conn1 : PMIOPort  Port=1  Side=Left
  Conn2 : PMIOPort  Port=2  Side=Right
  wires:
  Compare To Constant2/1 -> ON2/1
  Compare To Constat3/1 -> OFF2/1
  Clock4/1 -> Compare To Constat3/1, Compare To Constant2/1
  connections:
  OFF2/RConn1 -- Conn2/RConn1
  ON2/RConn1 -- OFF2/LConn1
  ON2/LConn1 -- Conn1/RConn1

== system Sim_Ideal/ON_OFF_12 ==
  Clock4 : Clock
  Compare To Constant2 : simulink/Logic and Bit Operations/Compare To Constant  relop=>=  const=sim_on(12)  OutDataTypeStr=boolean
  Compare To Constat3 : simulink/Logic and Bit Operations/Compare To Constant  relop=<=  const=sim_off(12)  OutDataTypeStr=boolean
  OFF2 : powerlib/Power Electronics/Ideal Switch  Ron=0.001  Lon=0  IC=0  Rs=1e5  Cs=inf  Measurements=off
  ON2 : powerlib/Power Electronics/Ideal Switch  Ron=0.001  Lon=0  IC=0  Rs=1e5  Cs=inf  Measurements=off
  Conn1 : PMIOPort  Port=1  Side=Left
  Conn2 : PMIOPort  Port=2  Side=Right
  wires:
  Compare To Constant2/1 -> ON2/1
  Compare To Constat3/1 -> OFF2/1
  Clock4/1 -> Compare To Constat3/1, Compare To Constant2/1
  connections:
  OFF2/RConn1 -- Conn2/RConn1
  ON2/RConn1 -- OFF2/LConn1
  ON2/LConn1 -- Conn1/RConn1

== system Sim_Ideal/ON_OFF_13 ==
  Clock6 : Clock
  Compare To Constant3 : simulink/Logic and Bit Operations/Compare To Constant  relop=>=  const=sim_on(13)  OutDataTypeStr=boolean
  Compare To Constat4 : simulink/Logic and Bit Operations/Compare To Constant  relop=<=  const=sim_off(13)  OutDataTypeStr=boolean
  OFF3 : powerlib/Power Electronics/Ideal Switch  Ron=0.001  Lon=0  IC=0  Rs=1e5  Cs=inf  Measurements=off
  ON3 : powerlib/Power Electronics/Ideal Switch  Ron=0.001  Lon=0  IC=0  Rs=1e5  Cs=inf  Measurements=off
  Conn1 : PMIOPort  Port=1  Side=Left
  Conn2 : PMIOPort  Port=2  Side=Right
  wires:
  Compare To Constant3/1 -> ON3/1
  Clock6/1 -> Compare To Constat4/1, Compare To Constant3/1
  Compare To Constat4/1 -> OFF3/1
  connections:
  ON3/RConn1 -- OFF3/LConn1
  OFF3/RConn1 -- Conn2/RConn1
  ON3/LConn1 -- Conn1/RConn1

== system Sim_Ideal/ON_OFF_14 ==
  Clock6 : Clock
  Compare To Constant3 : simulink/Logic and Bit Operations/Compare To Constant  relop=>=  const=sim_on(14)  OutDataTypeStr=boolean
  Compare To Constat4 : simulink/Logic and Bit Operations/Compare To Constant  relop=<=  const=sim_off(14)  OutDataTypeStr=boolean
  OFF3 : powerlib/Power Electronics/Ideal Switch  Ron=0.001  Lon=0  IC=0  Rs=1e5  Cs=inf  Measurements=off
  ON3 : powerlib/Power Electronics/Ideal Switch  Ron=0.001  Lon=0  IC=0  Rs=1e5  Cs=inf  Measurements=off
  Conn1 : PMIOPort  Port=1  Side=Left
  Conn2 : PMIOPort  Port=2  Side=Right
  wires:
  Compare To Constant3/1 -> ON3/1
  Clock6/1 -> Compare To Constat4/1, Compare To Constant3/1
  Compare To Constat4/1 -> OFF3/1
  connections:
  ON3/RConn1 -- OFF3/LConn1
  OFF3/RConn1 -- Conn2/RConn1
  ON3/LConn1 -- Conn1/RConn1

== system Sim_Ideal/ON_OFF_15 ==
  Clock6 : Clock
  Compare To Constant3 : simulink/Logic and Bit Operations/Compare To Constant  relop=>=  const=sim_on(15)  OutDataTypeStr=boolean
  Compare To Constat4 : simulink/Logic and Bit Operations/Compare To Constant  relop=<=  const=sim_off(15)  OutDataTypeStr=boolean
  OFF3 : powerlib/Power Electronics/Ideal Switch  Ron=0.001  Lon=0  IC=0  Rs=1e5  Cs=inf  Measurements=off
  ON3 : powerlib/Power Electronics/Ideal Switch  Ron=0.001  Lon=0  IC=0  Rs=1e5  Cs=inf  Measurements=off
  Conn1 : PMIOPort  Port=1  Side=Left
  Conn2 : PMIOPort  Port=2  Side=Right
  wires:
  Compare To Constant3/1 -> ON3/1
  Clock6/1 -> Compare To Constat4/1, Compare To Constant3/1
  Compare To Constat4/1 -> OFF3/1
  connections:
  ON3/RConn1 -- OFF3/LConn1
  OFF3/RConn1 -- Conn2/RConn1
  ON3/LConn1 -- Conn1/RConn1

== system Sim_Ideal/ON_OFF_16 ==
  Clock6 : Clock
  Compare To Constant3 : simulink/Logic and Bit Operations/Compare To Constant  relop=>=  const=sim_on(16)  OutDataTypeStr=boolean
  Compare To Constat4 : simulink/Logic and Bit Operations/Compare To Constant  relop=<=  const=sim_off(16)  OutDataTypeStr=boolean
  OFF3 : powerlib/Power Electronics/Ideal Switch  Ron=0.001  Lon=0  IC=0  Rs=1e5  Cs=inf  Measurements=off
  ON3 : powerlib/Power Electronics/Ideal Switch  Ron=0.001  Lon=0  IC=0  Rs=1e5  Cs=inf  Measurements=off
  Conn1 : PMIOPort  Port=1  Side=Left
  Conn2 : PMIOPort  Port=2  Side=Right
  wires:
  Compare To Constant3/1 -> ON3/1
  Clock6/1 -> Compare To Constat4/1, Compare To Constant3/1
  Compare To Constat4/1 -> OFF3/1
  connections:
  ON3/RConn1 -- OFF3/LConn1
  OFF3/RConn1 -- Conn2/RConn1
  ON3/LConn1 -- Conn1/RConn1

== system Sim_Ideal/ON_OFF_17 ==
  Clock7 : Clock
  Compare To Constant4 : simulink/Logic and Bit Operations/Compare To Constant  relop=>=  const=sim_on(17)  OutDataTypeStr=boolean
  Compare To Constat5 : simulink/Logic and Bit Operations/Compare To Constant  relop=<=  const=sim_off(17)  OutDataTypeStr=boolean
  OFF4 : powerlib/Power Electronics/Ideal Switch  Ron=0.001  Lon=0  IC=0  Rs=1e5  Cs=inf  Measurements=off
  ON4 : powerlib/Power Electronics/Ideal Switch  Ron=0.001  Lon=0  IC=0  Rs=1e5  Cs=inf  Measurements=off
  Conn1 : PMIOPort  Port=1  Side=Left
  Conn2 : PMIOPort  Port=2  Side=Right
  wires:
  Compare To Constat5/1 -> OFF4/1
  Clock7/1 -> Compare To Constat5/1, Compare To Constant4/1
  Compare To Constant4/1 -> ON4/1
  connections:
  ON4/RConn1 -- OFF4/LConn1
  OFF4/RConn1 -- Conn2/RConn1
  ON4/LConn1 -- Conn1/RConn1

== system Sim_Ideal/ON_OFF_18 ==
  Clock7 : Clock
  Compare To Constant4 : simulink/Logic and Bit Operations/Compare To Constant  relop=>=  const=sim_on(18)  OutDataTypeStr=boolean
  Compare To Constat5 : simulink/Logic and Bit Operations/Compare To Constant  relop=<=  const=sim_off(18)  OutDataTypeStr=boolean
  OFF4 : powerlib/Power Electronics/Ideal Switch  Ron=0.001  Lon=0  IC=0  Rs=1e5  Cs=inf  Measurements=off
  ON4 : powerlib/Power Electronics/Ideal Switch  Ron=0.001  Lon=0  IC=0  Rs=1e5  Cs=inf  Measurements=off
  Conn1 : PMIOPort  Port=1  Side=Left
  Conn2 : PMIOPort  Port=2  Side=Right
  wires:
  Compare To Constat5/1 -> OFF4/1
  Clock7/1 -> Compare To Constat5/1, Compare To Constant4/1
  Compare To Constant4/1 -> ON4/1
  connections:
  ON4/RConn1 -- OFF4/LConn1
  OFF4/RConn1 -- Conn2/RConn1
  ON4/LConn1 -- Conn1/RConn1

== system Sim_Ideal/ON_OFF_19 ==
  Clock7 : Clock
  Compare To Constant4 : simulink/Logic and Bit Operations/Compare To Constant  relop=>=  const=sim_on(19)  OutDataTypeStr=boolean
  Compare To Constat5 : simulink/Logic and Bit Operations/Compare To Constant  relop=<=  const=sim_off(19)  OutDataTypeStr=boolean
  OFF4 : powerlib/Power Electronics/Ideal Switch  Ron=0.001  Lon=0  IC=0  Rs=1e5  Cs=inf  Measurements=off
  ON4 : powerlib/Power Electronics/Ideal Switch  Ron=0.001  Lon=0  IC=0  Rs=1e5  Cs=inf  Measurements=off
  Conn1 : PMIOPort  Port=1  Side=Left
  Conn2 : PMIOPort  Port=2  Side=Right
  wires:
  Compare To Constat5/1 -> OFF4/1
  Clock7/1 -> Compare To Constat5/1, Compare To Constant4/1
  Compare To Constant4/1 -> ON4/1
  connections:
  ON4/RConn1 -- OFF4/LConn1
  OFF4/RConn1 -- Conn2/RConn1
  ON4/LConn1 -- Conn1/RConn1

== system Sim_Ideal/ON_OFF_2 ==
  Clock1 : Clock
  Clock2 : Clock
  Clock3 : Clock
  Compare To Constant : simulink/Logic and Bit Operations/Compare To Constant  relop=>=  const=sim_on(2)  OutDataTypeStr=boolean
  Compare To Constant1 : simulink/Logic and Bit Operations/Compare To Constant  relop=>=  const=sim_off(2)  OutDataTypeStr=boolean
  Compare To Constant2 : simulink/Logic and Bit Operations/Compare To Constant  relop=>=  const=sim_on(2)  OutDataTypeStr=boolean
  Constant : Constant  Value=0
  Constant1 : Constant  Value=0
  Ideal Switch : powerlib/Power Electronics/Ideal Switch  Ron=0.001  Lon=0  IC=0  Rs=1e5  Cs=inf  Measurements=off
  Switch : Switch
  Switch1 : Switch
  Conn1 : PMIOPort  Port=1  Side=Left
  Conn2 : PMIOPort  Port=2  Side=Left
  tag scope: tensao_2=global
  wires:
  Switch1/1 -> [tensao_2]
  Constant/1 -> Switch/3
  Switch/1 -> Switch1/3
  Clock1/1 -> Compare To Constant/1
  Clock2/1 -> Compare To Constant1/1
  Compare To Constant1/1 -> Switch1/2
  [fonte_tensao] -> Switch/1
  Constant1/1 -> Switch1/1
  Compare To Constant/1 -> Switch/2
  Clock3/1 -> Compare To Constant2/1
  Compare To Constant2/1 -> Ideal Switch/1
  connections:
  Conn1/RConn1 -- Ideal Switch/LConn1
  Ideal Switch/RConn1 -- Conn2/RConn1

== system Sim_Ideal/ON_OFF_20 ==
  Clock7 : Clock
  Compare To Constant4 : simulink/Logic and Bit Operations/Compare To Constant  relop=>=  const=sim_on(20)  OutDataTypeStr=boolean
  Compare To Constat5 : simulink/Logic and Bit Operations/Compare To Constant  relop=<=  const=sim_off(20)  OutDataTypeStr=boolean
  OFF4 : powerlib/Power Electronics/Ideal Switch  Ron=0.001  Lon=0  IC=0  Rs=1e5  Cs=inf  Measurements=off
  ON4 : powerlib/Power Electronics/Ideal Switch  Ron=0.001  Lon=0  IC=0  Rs=1e5  Cs=inf  Measurements=off
  Conn1 : PMIOPort  Port=1  Side=Left
  Conn2 : PMIOPort  Port=2  Side=Right
  wires:
  Compare To Constat5/1 -> OFF4/1
  Clock7/1 -> Compare To Constat5/1, Compare To Constant4/1
  Compare To Constant4/1 -> ON4/1
  connections:
  ON4/RConn1 -- OFF4/LConn1
  OFF4/RConn1 -- Conn2/RConn1
  ON4/LConn1 -- Conn1/RConn1

== system Sim_Ideal/ON_OFF_21 ==
  Clock8 : Clock
  Compare To Constant5 : simulink/Logic and Bit Operations/Compare To Constant  relop=>=  const=sim_on(21)  OutDataTypeStr=boolean
  Compare To Constat6 : simulink/Logic and Bit Operations/Compare To Constant  relop=<=  const=sim_off(21)  OutDataTypeStr=boolean
  OFF5 : powerlib/Power Electronics/Ideal Switch  Ron=0.001  Lon=0  IC=0  Rs=1e5  Cs=inf  Measurements=off
  ON5 : powerlib/Power Electronics/Ideal Switch  Ron=0.001  Lon=0  IC=0  Rs=1e5  Cs=inf  Measurements=off
  Conn1 : PMIOPort  Port=1  Side=Left
  Conn2 : PMIOPort  Port=2  Side=Right
  wires:
  Clock8/1 -> Compare To Constat6/1, Compare To Constant5/1
  Compare To Constat6/1 -> OFF5/1
  Compare To Constant5/1 -> ON5/1
  connections:
  ON5/RConn1 -- OFF5/LConn1
  OFF5/RConn1 -- Conn2/RConn1
  ON5/LConn1 -- Conn1/RConn1

== system Sim_Ideal/ON_OFF_22 ==
  Clock8 : Clock
  Compare To Constant5 : simulink/Logic and Bit Operations/Compare To Constant  relop=>=  const=sim_on(22)  OutDataTypeStr=boolean
  Compare To Constat6 : simulink/Logic and Bit Operations/Compare To Constant  relop=<=  const=sim_off(22)  OutDataTypeStr=boolean
  OFF5 : powerlib/Power Electronics/Ideal Switch  Ron=0.001  Lon=0  IC=0  Rs=1e5  Cs=inf  Measurements=off
  ON5 : powerlib/Power Electronics/Ideal Switch  Ron=0.001  Lon=0  IC=0  Rs=1e5  Cs=inf  Measurements=off
  Conn1 : PMIOPort  Port=1  Side=Left
  Conn2 : PMIOPort  Port=2  Side=Right
  wires:
  Clock8/1 -> Compare To Constat6/1, Compare To Constant5/1
  Compare To Constat6/1 -> OFF5/1
  Compare To Constant5/1 -> ON5/1
  connections:
  ON5/RConn1 -- OFF5/LConn1
  OFF5/RConn1 -- Conn2/RConn1
  ON5/LConn1 -- Conn1/RConn1

== system Sim_Ideal/ON_OFF_23 ==
  Clock8 : Clock
  Compare To Constant5 : simulink/Logic and Bit Operations/Compare To Constant  relop=>=  const=sim_on(23)  OutDataTypeStr=boolean
  Compare To Constat6 : simulink/Logic and Bit Operations/Compare To Constant  relop=<=  const=sim_off(23)  OutDataTypeStr=boolean
  OFF5 : powerlib/Power Electronics/Ideal Switch  Ron=0.001  Lon=0  IC=0  Rs=1e5  Cs=inf  Measurements=off
  ON5 : powerlib/Power Electronics/Ideal Switch  Ron=0.001  Lon=0  IC=0  Rs=1e5  Cs=inf  Measurements=off
  Conn1 : PMIOPort  Port=1  Side=Left
  Conn2 : PMIOPort  Port=2  Side=Right
  wires:
  Clock8/1 -> Compare To Constat6/1, Compare To Constant5/1
  Compare To Constat6/1 -> OFF5/1
  Compare To Constant5/1 -> ON5/1
  connections:
  ON5/RConn1 -- OFF5/LConn1
  OFF5/RConn1 -- Conn2/RConn1
  ON5/LConn1 -- Conn1/RConn1

== system Sim_Ideal/ON_OFF_24 ==
  Clock8 : Clock
  Compare To Constant5 : simulink/Logic and Bit Operations/Compare To Constant  relop=>=  const=sim_on(24)  OutDataTypeStr=boolean
  Compare To Constat6 : simulink/Logic and Bit Operations/Compare To Constant  relop=<=  const=sim_off(24)  OutDataTypeStr=boolean
  OFF5 : powerlib/Power Electronics/Ideal Switch  Ron=0.001  Lon=0  IC=0  Rs=1e5  Cs=inf  Measurements=off
  ON5 : powerlib/Power Electronics/Ideal Switch  Ron=0.001  Lon=0  IC=0  Rs=1e5  Cs=inf  Measurements=off
  Conn1 : PMIOPort  Port=1  Side=Left
  Conn2 : PMIOPort  Port=2  Side=Right
  wires:
  Clock8/1 -> Compare To Constat6/1, Compare To Constant5/1
  Compare To Constat6/1 -> OFF5/1
  Compare To Constant5/1 -> ON5/1
  connections:
  ON5/RConn1 -- OFF5/LConn1
  OFF5/RConn1 -- Conn2/RConn1
  ON5/LConn1 -- Conn1/RConn1

== system Sim_Ideal/ON_OFF_25 ==
  Clock8 : Clock
  Compare To Constant5 : simulink/Logic and Bit Operations/Compare To Constant  relop=>=  const=sim_on(25)  OutDataTypeStr=boolean
  Compare To Constat6 : simulink/Logic and Bit Operations/Compare To Constant  relop=<=  const=sim_off(25)  OutDataTypeStr=boolean
  OFF5 : powerlib/Power Electronics/Ideal Switch  Ron=0.001  Lon=0  IC=0  Rs=1e5  Cs=inf  Measurements=off
  ON5 : powerlib/Power Electronics/Ideal Switch  Ron=0.001  Lon=0  IC=0  Rs=1e5  Cs=inf  Measurements=off
  Conn1 : PMIOPort  Port=1  Side=Left
  Conn2 : PMIOPort  Port=2  Side=Right
  wires:
  Clock8/1 -> Compare To Constat6/1, Compare To Constant5/1
  Compare To Constat6/1 -> OFF5/1
  Compare To Constant5/1 -> ON5/1
  connections:
  ON5/RConn1 -- OFF5/LConn1
  OFF5/RConn1 -- Conn2/RConn1
  ON5/LConn1 -- Conn1/RConn1

== system Sim_Ideal/ON_OFF_26 ==
  Clock8 : Clock
  Compare To Constant5 : simulink/Logic and Bit Operations/Compare To Constant  relop=>=  const=sim_on(26)  OutDataTypeStr=boolean
  Compare To Constat6 : simulink/Logic and Bit Operations/Compare To Constant  relop=<=  const=sim_off(26)  OutDataTypeStr=boolean
  OFF5 : powerlib/Power Electronics/Ideal Switch  Ron=0.001  Lon=0  IC=0  Rs=1e5  Cs=inf  Measurements=off
  ON5 : powerlib/Power Electronics/Ideal Switch  Ron=0.001  Lon=0  IC=0  Rs=1e5  Cs=inf  Measurements=off
  Conn1 : PMIOPort  Port=1  Side=Left
  Conn2 : PMIOPort  Port=2  Side=Right
  wires:
  Clock8/1 -> Compare To Constat6/1, Compare To Constant5/1
  Compare To Constat6/1 -> OFF5/1
  Compare To Constant5/1 -> ON5/1
  connections:
  ON5/RConn1 -- OFF5/LConn1
  OFF5/RConn1 -- Conn2/RConn1
  ON5/LConn1 -- Conn1/RConn1

== system Sim_Ideal/ON_OFF_27 ==
  Clock8 : Clock
  Compare To Constant5 : simulink/Logic and Bit Operations/Compare To Constant  relop=>=  const=sim_on(27)  OutDataTypeStr=boolean
  Compare To Constat6 : simulink/Logic and Bit Operations/Compare To Constant  relop=<=  const=sim_off(27)  OutDataTypeStr=boolean
  OFF5 : powerlib/Power Electronics/Ideal Switch  Ron=0.001  Lon=0  IC=0  Rs=1e5  Cs=inf  Measurements=off
  ON5 : powerlib/Power Electronics/Ideal Switch  Ron=0.001  Lon=0  IC=0  Rs=1e5  Cs=inf  Measurements=off
  Conn1 : PMIOPort  Port=1  Side=Left
  Conn2 : PMIOPort  Port=2  Side=Right
  wires:
  Clock8/1 -> Compare To Constat6/1, Compare To Constant5/1
  Compare To Constat6/1 -> OFF5/1
  Compare To Constant5/1 -> ON5/1
  connections:
  ON5/RConn1 -- OFF5/LConn1
  OFF5/RConn1 -- Conn2/RConn1
  ON5/LConn1 -- Conn1/RConn1

== system Sim_Ideal/ON_OFF_28 ==
  Clock8 : Clock
  Compare To Constant5 : simulink/Logic and Bit Operations/Compare To Constant  relop=>=  const=sim_on(28)  OutDataTypeStr=boolean
  Compare To Constat6 : simulink/Logic and Bit Operations/Compare To Constant  relop=<=  const=sim_off(28)  OutDataTypeStr=boolean
  OFF5 : powerlib/Power Electronics/Ideal Switch  Ron=0.001  Lon=0  IC=0  Rs=1e5  Cs=inf  Measurements=off
  ON5 : powerlib/Power Electronics/Ideal Switch  Ron=0.001  Lon=0  IC=0  Rs=1e5  Cs=inf  Measurements=off
  Conn1 : PMIOPort  Port=1  Side=Left
  Conn2 : PMIOPort  Port=2  Side=Right
  wires:
  Clock8/1 -> Compare To Constat6/1, Compare To Constant5/1
  Compare To Constat6/1 -> OFF5/1
  Compare To Constant5/1 -> ON5/1
  connections:
  ON5/RConn1 -- OFF5/LConn1
  OFF5/RConn1 -- Conn2/RConn1
  ON5/LConn1 -- Conn1/RConn1

== system Sim_Ideal/ON_OFF_3 ==
  Clock1 : Clock
  Clock2 : Clock
  Clock3 : Clock
  Compare To Constant : simulink/Logic and Bit Operations/Compare To Constant  relop=>=  const=sim_on(3)  OutDataTypeStr=boolean
  Compare To Constant1 : simulink/Logic and Bit Operations/Compare To Constant  relop=>=  const=sim_off(3)  OutDataTypeStr=boolean
  Compare To Constant2 : simulink/Logic and Bit Operations/Compare To Constant  relop=>=  const=sim_on(3)  OutDataTypeStr=boolean
  Constant : Constant  Value=0
  Constant1 : Constant  Value=0
  Ideal Switch : powerlib/Power Electronics/Ideal Switch  Ron=0.001  Lon=0  IC=0  Rs=1e5  Cs=inf  Measurements=off
  Switch : Switch
  Switch1 : Switch
  Conn1 : PMIOPort  Port=1  Side=Left
  Conn2 : PMIOPort  Port=2  Side=Left
  tag scope: tensao_3=global
  wires:
  Switch1/1 -> [tensao_3]
  Constant/1 -> Switch/3
  Switch/1 -> Switch1/3
  Clock1/1 -> Compare To Constant/1
  Clock2/1 -> Compare To Constant1/1
  Compare To Constant1/1 -> Switch1/2
  [fonte_tensao] -> Switch/1
  Constant1/1 -> Switch1/1
  Compare To Constant/1 -> Switch/2
  Clock3/1 -> Compare To Constant2/1
  Compare To Constant2/1 -> Ideal Switch/1
  connections:
  Conn1/RConn1 -- Ideal Switch/LConn1
  Ideal Switch/RConn1 -- Conn2/RConn1

== system Sim_Ideal/ON_OFF_4 ==
  Clock1 : Clock
  Clock2 : Clock
  Clock3 : Clock
  Compare To Constant : simulink/Logic and Bit Operations/Compare To Constant  relop=>=  const=sim_on(4)  OutDataTypeStr=boolean
  Compare To Constant1 : simulink/Logic and Bit Operations/Compare To Constant  relop=>=  const=sim_off(4)  OutDataTypeStr=boolean
  Compare To Constant2 : simulink/Logic and Bit Operations/Compare To Constant  relop=>=  const=sim_on(4)  OutDataTypeStr=boolean
  Constant : Constant  Value=0
  Constant1 : Constant  Value=0
  Ideal Switch : powerlib/Power Electronics/Ideal Switch  Ron=0.001  Lon=0  IC=0  Rs=1e5  Cs=inf  Measurements=off
  Switch : Switch
  Switch1 : Switch
  Conn1 : PMIOPort  Port=1  Side=Left
  Conn2 : PMIOPort  Port=2  Side=Left
  tag scope: tensao_4=global
  wires:
  Switch1/1 -> [tensao_4]
  Constant/1 -> Switch/3
  Switch/1 -> Switch1/3
  Clock1/1 -> Compare To Constant/1
  Clock2/1 -> Compare To Constant1/1
  Compare To Constant1/1 -> Switch1/2
  [fonte_tensao] -> Switch/1
  Constant1/1 -> Switch1/1
  Compare To Constant/1 -> Switch/2
  Clock3/1 -> Compare To Constant2/1
  Compare To Constant2/1 -> Ideal Switch/1
  connections:
  Conn1/RConn1 -- Ideal Switch/LConn1
  Ideal Switch/RConn1 -- Conn2/RConn1

== system Sim_Ideal/ON_OFF_5 ==
  Clock1 : Clock
  Compare To Constant1 : simulink/Logic and Bit Operations/Compare To Constant  relop=>=  const=sim_on(5)  OutDataTypeStr=boolean
  Compare To Constat1 : simulink/Logic and Bit Operations/Compare To Constant  relop=<=  const=sim_off(5)  OutDataTypeStr=boolean
  OFF1 : powerlib/Power Electronics/Ideal Switch  Ron=0.001  Lon=0  IC=0  Rs=1e5  Cs=inf  Measurements=off
  ON1 : powerlib/Power Electronics/Ideal Switch  Ron=0.001  Lon=0  IC=0  Rs=1e5  Cs=inf  Measurements=off
  Conn1 : PMIOPort  Port=1  Side=Left
  Conn2 : PMIOPort  Port=2  Side=Right
  wires:
  Compare To Constat1/1 -> OFF1/1
  Compare To Constant1/1 -> ON1/1
  Clock1/1 -> Compare To Constat1/1, Compare To Constant1/1
  connections:
  ON1/RConn1 -- OFF1/LConn1
  Conn1/RConn1 -- ON1/LConn1
  OFF1/RConn1 -- Conn2/RConn1
